simulink model "myrobot"  (R2019b)
settings: Solver=FixedStepAuto  StartTime=0.0  StopTime=2  FixedStep=0.001  MaxStep=0.005  RelTol=1e-3
undefined symbols (not defined in the file or in its folder): X, Y, Z
libraries: sm_lib x17, nesl_utility x13, robotmaniplib x4, simulink x2
(part 6 of 7)

== matlab function myrobot/TRAJECTORY GENERATION/MATLAB Function2 ==
  data: X output; Y output; Z output; T output; t input
function [X, Y, Z, T]  = trajectory_generator(t)

t = 0.1;
X = 0.3 + 0.2 * cos(5*pi*t);
Y = 0.45;
Z = 0.3 + 0.2 * sin(5*pi*t);

T = [1 0 0 X;
     0 1 0 Y;
     0 0 1 Z;
     0 0 0 1];

end

== matlab function myrobot/MATLAB Function ==
  data: q input; X output; Y output; Z output
function [X, Y, Z] = FK(q)

T_01 = [1 0 0 0;
        0 1 0 0;
        0 0 1 0.07;
        0 0 0 1]; 

T_1dot2 = [0 0 1 0.08;
           1 0 0 0;
           0 1 0 0.12;
           0 0 0 1];

T_2dot3 = [1 0 0 0;
           0 1 0 0.43;
           0 0 1 0;
           0 0 0 1];

T_3dot4 = [0 -1 0 0;
           0 0 1 0.335;
           -1 0 0 -0.08;
           0 0 0 1];

T_11dot = [cos(q(1)) -sin(q(1)) 0 0;
           sin(q(1)) cos(q(1)) 0 0;
           0 0 1 0
           0 0 0 1];

T_22dot = [cos(q(2)) -sin(q(2)) 0 0;
           sin(q(2)) cos(q(2)) 0 0;
           0 0 1 0
           0 0 0 1];

T_33dot = [cos(q(3)) -sin(q(3)) 0 0;
           sin(q(3)) cos(q(3)) 0 0;
           0 0 1 0
           0 0 0 1];

T_01dot = T_01 * T_11dot;
T_02dot = T_01dot * T_1dot2 * T_22dot;
T_03dot = T_02dot * T_2dot3 * T_33dot;
T_0EE = T_03dot * T_3dot4;


X = T_0EE(1,4);
Y = T_0EE(2,4);
Z = T_0EE(3,4);

end

== matlab function myrobot/MATLAB Function2 ==
  data: output output; q input; q_dot input; q_ddot input
function output = linear_parameterized(q, q_dot, q_ddot)

g = 9.81;

Y = [ q_dot(1)*q_dot(2)*sin(2*q(2)) - q_ddot(1)*(cos(2*q(2))/2 - 1/2), q_ddot(1)*sin(2*q(2)) + 2*q_dot(1)*q_dot(2)*cos(2*q(2)), q_dot(1)*((q_dot(2)*sin(2*q(2) + 2*q(3)))/2 + (q_dot(3)*sin(2*q(2) + 2*q(3)))/2) - q_ddot(1)*(cos(2*q(2) + 2*q(3))/2 - 1/2) + (q_dot(1)*q_dot(2)*sin(2*q(2) + 2*q(3)))/2 + (q_dot(1)*q_dot(3)*sin(2*q(2) + 2*q(3)))/2, q_ddot(1)*(cos(2*q(2))/2 + 1/2) - q_dot(1)*q_dot(2)*sin(2*q(2)), cos(q(2))*q_dot(2)^2 + q_ddot(2)*sin(q(2)), q_ddot(1)*sin(2*q(2) + 2*q(3)) + q_dot(1)*(q_dot(2)*cos(2*q(2) + 2*q(3)) + q_dot(3)*cos(2*q(2) + 2*q(3))) + q_dot(1)*q_dot(2)*cos(2*q(2) + 2*q(3)) + q_dot(1)*q_dot(3)*cos(2*q(2) + 2*q(3)), q_ddot(1), - sin(q(2))*q_dot(2)^2 + q_ddot(2)*cos(q(2)), q_ddot(1)*(cos(2*q(2) + 2*q(3))/2 + 1/2) - q_dot(1)*((q_dot(2)*sin(2*q(2) + 2*q(3)))/2 + (q_dot(3)*sin(2*q(2) + 2*q(3)))/2) - (q_dot(1)*q_dot(2)*sin(2*q(2) + 2*q(3)))/2 - (q_dot(1)*q_dot(3)*sin(2*q(2) + 2*q(3)))/2, q_dot(2)*(q_dot(2)*cos(q(2) + q(3)) + q_dot(3)*cos(q(2) + q(3))) + q_dot(3)*(q_dot(2)*cos(q(2) + q(3)) + q_dot(3)*cos(q(2) + q(3))) + q_ddot(2)*sin(q(2) + q(3)) + q_ddot(3)*sin(q(2) + q(3)),           0, q_ddot(2)*cos(q(2) + q(3)) - q_dot(3)*(q_dot(2)*sin(q(2) + q(3)) + q_dot(3)*sin(q(2) + q(3))) - q_dot(2)*(q_dot(2)*sin(q(2) + q(3)) + q_dot(3)*sin(q(2) + q(3))) + q_ddot(3)*cos(q(2) + q(3)),                         0,              0,              0,                       0, q_ddot(1), q_ddot(1), q_dot(1)*q_dot(2)*sin(2*q(2)) - q_ddot(1)*(cos(2*q(2))/2 - 1/2), q_ddot(1), q_dot(1)*q_dot(2)*sin(2*q(2)) - q_ddot(1)*(cos(2*q(2))/2 - 1/2), q_ddot(1), q_dot(1)*((q_dot(2)*sin(2*q(2) + 2*q(3)))/2 + (q_dot(3)*sin(2*q(2) + 2*q(3)))/2) - q_ddot(1)*(cos(2*q(2) + 2*q(3))/2 - 1/2) + (q_dot(1)*q_dot(2)*sin(2*q(2) + 2*q(3)))/2 + (q_dot(1)*q_dot(3)*sin(2*q(2) + 2*q(3)))/2, q_ddot(1), sin(q(2))*q_dot(2)^2 - q_ddot(2)*cos(q(2)), sin(q(2))*q_dot(2)^2 - q_ddot(2)*cos(q(2)), 2*q_ddot(1), q_dot(2)*(q_dot(2)*sin(q(2) + q(3)) + q_dot(3)*sin(q(2) + q(3))) + q_dot(3)*(q_dot(2)*sin(q(2) + q(3)) + q_dot(3)*sin(q(2) + q(3))) - q_ddot(2)*cos(q(2) + q(3)) - q_ddot(3)*cos(q(2) + q(3)), 2*q_ddot(1), q_dot(1)*(q_dot(2)*sin(2*q(2) + q(3)) + q_dot(3)*(sin(2*q(2) + q(3))/2 - sin(q(3))/2)) - q_ddot(1)*(cos(2*q(2) + q(3)) - cos(q(3))) - q_dot(3)*((q_dot(1)*sin(q(3)))/2 - (q_dot(1)*sin(2*q(2) + q(3)))/2) + q_dot(1)*q_dot(2)*sin(2*q(2) + q(3)), sin(q(2))*q_dot(2)^2 - q_ddot(2)*cos(q(2)), sin(q(2))*q_dot(2)^2 - q_ddot(2)*cos(q(2)), q_dot(2)*(q_dot(2)*sin(q(2) + q(3)) + q_dot(3)*sin(q(2) + q(3))) + q_dot(3)*(q_dot(2)*sin(q(2) + q(3)) + q_dot(3)*sin(q(2) + q(3))) - q_ddot(2)*cos(q(2) + q(3)) - q_ddot(3)*cos(q(2) + q(3));
                                           -(q_dot(1)^2*sin(2*q(2)))/2,                                       -q_dot(1)^2*cos(2*q(2)),                                                                                                                                                                                                                -(q_dot(1)^2*sin(2*q(2) + 2*q(3)))/2,                                            (q_dot(1)^2*sin(2*q(2)))/2,                            q_ddot(1)*sin(q(2)),                                                                                                                                                                                          -q_dot(1)^2*cos(2*q(2) + 2*q(3)),           0,                              q_ddot(1)*cos(q(2)),                                                                                                                                                                                                                 (q_dot(1)^2*sin(2*q(2) + 2*q(3)))/2,                                                                                                                                                                                                      q_ddot(1)*sin(q(2) + q(3)), q_ddot(2),                                                                                                                                                                                                      q_ddot(1)*cos(q(2) + q(3)), q_ddot(2) + q_ddot(3), -g*sin(q(2)), -g*sin(q(2)), -g*sin(q(2) + q(3)),           0,           0,                              q_ddot(2) - (q_dot(1)^2*sin(2*q(2)))/2,           0,                              q_ddot(2) - (q_dot(1)^2*sin(2*q(2)))/2,           0,                                                                                                                                                                                     q_ddot(2) + q_ddot(3) - (q_dot(1)^2*sin(2*q(2) + 2*q(3)))/2,           0,                           -q_ddot(1)*cos(q(2)),                           -q_ddot(1)*cos(q(2)),             0,                                                                                                                                                                                                     -q_ddot(1)*cos(q(2) + q(3)),             0,                                                                                                           - sin(2*q(2) + q(3))*q_dot(1)^2 + 2*q_ddot(2)*cos(q(3)) + q_ddot(3)*cos(q(3)) - q_dot(3)*sin(q(3))*(q_dot(2) + q_dot(3)) - q_dot(2)*q_dot(3)*sin(q(3)),                           -q_ddot(1)*cos(q(2)),                           -q_ddot(1)*cos(q(2)),                                                                                                                                                                                                     -q_ddot(1)*cos(q(2) + q(3));
                                                                         0,                                                                 0,                                                                                                                                                                                                                -(q_dot(1)^2*sin(2*q(2) + 2*q(3)))/2,                                                                         0,                                                  0,                                                                                                                                                                                          -q_dot(1)^2*cos(2*q(2) + 2*q(3)),           0,                                                    0,                                                                                                                                                                                                                 (q_dot(1)^2*sin(2*q(2) + 2*q(3)))/2,                                                                                                                                                                                                      q_ddot(1)*sin(q(2) + q(3)),           0,                                                                                                                                                                                                      q_ddot(1)*cos(q(2) + q(3)), q_ddot(2) + q_ddot(3),              0,              0, -g*sin(q(2) + q(3)),           0,           0,                                                                         0,           0,                                                                         0,           0,                                                                                                                                                                                     q_ddot(2) + q_ddot(3) - (q_dot(1)^2*sin(2*q(2) + 2*q(3)))/2,           0,                                                  0,                                                  0,             0,                                                                                                                                                                                                     -q_ddot(1)*cos(q(2) + q(3)),             0,                                                                                                                                                                                 (sin(q(3))/2 - sin(2*q(2) + q(3))/2)*q_dot(1)^2 + sin(q(3))*q_dot(2)^2 + q_ddot(2)*cos(q(3)),                                                  0,                                                  0,                                                                                                                                                                                                     -q_ddot(1)*cos(q(2) + q(3))];

THETA = [0.253740000000000,1.41285000000000e-07,0.0754340000000000,0.0212824000000000,-7.13886000000000e-08,2.67415000000000e-08,0.00604953000000000,0.00499483000000000,0.0104250000000000,2.13561000000000e-09,0.247523000000000,0.00274946000000000,0.0744749000000000,2.21400980000000,1.73854678600000,0.622883338500000,0.0521152000000000,0.0329527040000000,0.952024214000000,0.000192286280344500,0.371183215904572,0.0688146654633342,0.0753533118750375,0.0294165347194417,0.177120784000000,0.139083742880000,0.0598856414640000,0.0498306670800000,-0.0311344561750400,0.267839835555000,-0.167347701940840,0.159821302798087,-0.0470811354471933];

output = Y * THETA';

end

== matlab function myrobot/VERIFYING PASSIVITY PARAMETER LINEARIZATION/MATLAB Function1 ==
  data: q input; output output; q_dot input; a input; v input
function output = passivity_linear_parameterized(q, q_dot, a, v)

g = 9.81;

Y = [ (q_dot(1)*v(2)*sin(2*q(2)))/2 - a(1)*(cos(2*q(2))/2 - 1/2) + (q_dot(2)*v(1)*sin(2*q(2)))/2, a(1)*sin(2*q(2)) + q_dot(1)*v(2)*cos(2*q(2)) + q_dot(2)*v(1)*cos(2*q(2)), v(1)*((q_dot(2)*sin(2*q(2) + 2*q(3)))/2 + (q_dot(3)*sin(2*q(2) + 2*q(3)))/2) - a(1)*(cos(2*q(2) + 2*q(3))/2 - 1/2) + (q_dot(1)*v(2)*sin(2*q(2) + 2*q(3)))/2 + (q_dot(1)*v(3)*sin(2*q(2) + 2*q(3)))/2, a(1)*(cos(2*q(2))/2 + 1/2) - (q_dot(1)*v(2)*sin(2*q(2)))/2 - (q_dot(2)*v(1)*sin(2*q(2)))/2, a(2)*sin(q(2)) + q_dot(2)*v(2)*cos(q(2)), a(1)*sin(2*q(2) + 2*q(3)) + v(1)*(q_dot(2)*cos(2*q(2) + 2*q(3)) + q_dot(3)*cos(2*q(2) + 2*q(3))) + q_dot(1)*v(2)*cos(2*q(2) + 2*q(3)) + q_dot(1)*v(3)*cos(2*q(2) + 2*q(3)), a(1), a(2)*cos(q(2)) - q_dot(2)*v(2)*sin(q(2)), a(1)*(cos(2*q(2) + 2*q(3))/2 + 1/2) - v(1)*((q_dot(2)*sin(2*q(2) + 2*q(3)))/2 + (q_dot(3)*sin(2*q(2) + 2*q(3)))/2) - (q_dot(1)*v(2)*sin(2*q(2) + 2*q(3)))/2 - (q_dot(1)*v(3)*sin(2*q(2) + 2*q(3)))/2, v(2)*(q_dot(2)*cos(q(2) + q(3)) + q_dot(3)*cos(q(2) + q(3))) + v(3)*(q_dot(2)*cos(q(2) + q(3)) + q_dot(3)*cos(q(2) + q(3))) + a(2)*sin(q(2) + q(3)) + a(3)*sin(q(2) + q(3)),  0, a(2)*cos(q(2) + q(3)) - v(3)*(q_dot(2)*sin(q(2) + q(3)) + q_dot(3)*sin(q(2) + q(3))) - v(2)*(q_dot(2)*sin(q(2) + q(3)) + q_dot(3)*sin(q(2) + q(3))) + a(3)*cos(q(2) + q(3)),       0,              0,              0,                       0, a(1), a(1), (q_dot(1)*v(2)*sin(2*q(2)))/2 - a(1)*(cos(2*q(2))/2 - 1/2) + (q_dot(2)*v(1)*sin(2*q(2)))/2, a(1), (q_dot(1)*v(2)*sin(2*q(2)))/2 - a(1)*(cos(2*q(2))/2 - 1/2) + (q_dot(2)*v(1)*sin(2*q(2)))/2, a(1), v(1)*((q_dot(2)*sin(2*q(2) + 2*q(3)))/2 + (q_dot(3)*sin(2*q(2) + 2*q(3)))/2) - a(1)*(cos(2*q(2) + 2*q(3))/2 - 1/2) + (q_dot(1)*v(2)*sin(2*q(2) + 2*q(3)))/2 + (q_dot(1)*v(3)*sin(2*q(2) + 2*q(3)))/2, a(1), q_dot(2)*v(2)*sin(q(2)) - a(2)*cos(q(2)), q_dot(2)*v(2)*sin(q(2)) - a(2)*cos(q(2)), 2*a(1), v(2)*(q_dot(2)*sin(q(2) + q(3)) + q_dot(3)*sin(q(2) + q(3))) + v(3)*(q_dot(2)*sin(q(2) + q(3)) + q_dot(3)*sin(q(2) + q(3))) - a(2)*cos(q(2) + q(3)) - a(3)*cos(q(2) + q(3)), 2*a(1), v(1)*(q_dot(2)*sin(2*q(2) + q(3)) + q_dot(3)*(sin(2*q(2) + q(3))/2 - sin(q(3))/2)) - a(1)*(cos(2*q(2) + q(3)) - cos(q(3))) - v(3)*((q_dot(1)*sin(q(3)))/2 - (q_dot(1)*sin(2*q(2) + q(3)))/2) + q_dot(1)*v(2)*sin(2*q(2) + q(3)), q_dot(2)*v(2)*sin(q(2)) - a(2)*cos(q(2)), q_dot(2)*v(2)*sin(q(2)) - a(2)*cos(q(2)), v(2)*(q_dot(2)*sin(q(2) + q(3)) + q_dot(3)*sin(q(2) + q(3))) + v(3)*(q_dot(2)*sin(q(2) + q(3)) + q_dot(3)*sin(q(2) + q(3))) - a(2)*cos(q(2) + q(3)) - a(3)*cos(q(2) + q(3));
                                                               -(q_dot(1)*v(1)*sin(2*q(2)))/2,                                                 -q_dot(1)*v(1)*cos(2*q(2)),                                                                                                                                                                              -(q_dot(1)*v(1)*sin(2*q(2) + 2*q(3)))/2,                                                                (q_dot(1)*v(1)*sin(2*q(2)))/2,                             a(1)*sin(q(2)),                                                                                                                                                        -q_dot(1)*v(1)*cos(2*q(2) + 2*q(3)),  0,                             a(1)*cos(q(2)),                                                                                                                                                                               (q_dot(1)*v(1)*sin(2*q(2) + 2*q(3)))/2,                                                                                                                                                                             a(1)*sin(q(2) + q(3)), a(2),                                                                                                                                                                             a(1)*cos(q(2) + q(3)), a(2) + a(3), -g*sin(q(2)), -g*sin(q(2)), -g*sin(q(2) + q(3)),  0,  0,                                                           a(2) - (q_dot(1)*v(1)*sin(2*q(2)))/2,  0,                                                           a(2) - (q_dot(1)*v(1)*sin(2*q(2)))/2,  0,                                                                                                                                                                     a(2) + a(3) - (q_dot(1)*v(1)*sin(2*q(2) + 2*q(3)))/2,  0,                            -a(1)*cos(q(2)),                            -a(1)*cos(q(2)),    0,                                                                                                                                                                            -a(1)*cos(q(2) + q(3)),    0,                                                                                                             2*a(2)*cos(q(3)) + a(3)*cos(q(3)) - v(3)*sin(q(3))*(q_dot(2) + q_dot(3)) - q_dot(3)*v(2)*sin(q(3)) - q_dot(1)*v(1)*sin(2*q(2) + q(3)),                            -a(1)*cos(q(2)),                            -a(1)*cos(q(2)),                                                                                                                                                                            -a(1)*cos(q(2) + q(3));
                                                                                              0,                                                                            0,                                                                                                                                                                              -(q_dot(1)*v(1)*sin(2*q(2) + 2*q(3)))/2,                                                                                              0,                                          0,                                                                                                                                                        -q_dot(1)*v(1)*cos(2*q(2) + 2*q(3)),  0,                                          0,                                                                                                                                                                               (q_dot(1)*v(1)*sin(2*q(2) + 2*q(3)))/2,                                                                                                                                                                             a(1)*sin(q(2) + q(3)),  0,                                                                                                                                                                             a(1)*cos(q(2) + q(3)), a(2) + a(3),              0,              0, -g*sin(q(2) + q(3)),  0,  0,                                                                                              0,  0,                                                                                              0,  0,                                                                                                                                                                     a(2) + a(3) - (q_dot(1)*v(1)*sin(2*q(2) + 2*q(3)))/2,  0,                                          0,                                          0,    0,                                                                                                                                                                            -a(1)*cos(q(2) + q(3)),    0,                                                                                                                                                       a(2)*cos(q(3)) + q_dot(2)*v(2)*sin(q(3)) - q_dot(1)*v(1)*(sin(2*q(2) + q(3))/2 - sin(q(3))/2),                                          0,                                          0,                                                                                                                                                                            -a(1)*cos(q(2) + q(3))];
 
THETA = [0.253740000000000,1.41285000000000e-07,0.0754340000000000,0.0212824000000000,-7.13886000000000e-08,2.67415000000000e-08,0.00604953000000000,0.00499483000000000,0.0104250000000000,2.13561000000000e-09,0.247523000000000,0.00274946000000000,0.0744749000000000,2.21400980000000,1.73854678600000,0.622883338500000,0.0521152000000000,0.0329527040000000,0.952024214000000,0.000192286280344500,0.371183215904572,0.0688146654633342,0.0753533118750375,0.0294165347194417,0.177120784000000,0.139083742880000,0.0598856414640000,0.0498306670800000,-0.0311344561750400,0.267839835555000,-0.167347701940840,0.159821302798087,-0.0470811354471933];

output = Y * THETA';

end

== matlab function myrobot/JOINT SPACE PASSIVITY BASED ROBUST CONTROLLER/MATLAB Function3 ==
  data: q input; output output; q_dot input; a input; v input; delta_theta input
function output = robust_passivity_linear_parameterized(q, q_dot, a, v, delta_theta)

g = 9.81;

Y = [ (q_dot(1)*v(2)*sin(2*q(2)))/2 - a(1)*(cos(2*q(2))/2 - 1/2) + (q_dot(2)*v(1)*sin(2*q(2)))/2, a(1)*sin(2*q(2)) + q_dot(1)*v(2)*cos(2*q(2)) + q_dot(2)*v(1)*cos(2*q(2)), v(1)*((q_dot(2)*sin(2*q(2) + 2*q(3)))/2 + (q_dot(3)*sin(2*q(2) + 2*q(3)))/2) - a(1)*(cos(2*q(2) + 2*q(3))/2 - 1/2) + (q_dot(1)*v(2)*sin(2*q(2) + 2*q(3)))/2 + (q_dot(1)*v(3)*sin(2*q(2) + 2*q(3)))/2, a(1)*(cos(2*q(2))/2 + 1/2) - (q_dot(1)*v(2)*sin(2*q(2)))/2 - (q_dot(2)*v(1)*sin(2*q(2)))/2, a(2)*sin(q(2)) + q_dot(2)*v(2)*cos(q(2)), a(1)*sin(2*q(2) + 2*q(3)) + v(1)*(q_dot(2)*cos(2*q(2) + 2*q(3)) + q_dot(3)*cos(2*q(2) + 2*q(3))) + q_dot(1)*v(2)*cos(2*q(2) + 2*q(3)) + q_dot(1)*v(3)*cos(2*q(2) + 2*q(3)), a(1), a(2)*cos(q(2)) - q_dot(2)*v(2)*sin(q(2)), a(1)*(cos(2*q(2) + 2*q(3))/2 + 1/2) - v(1)*((q_dot(2)*sin(2*q(2) + 2*q(3)))/2 + (q_dot(3)*sin(2*q(2) + 2*q(3)))/2) - (q_dot(1)*v(2)*sin(2*q(2) + 2*q(3)))/2 - (q_dot(1)*v(3)*sin(2*q(2) + 2*q(3)))/2, v(2)*(q_dot(2)*cos(q(2) + q(3)) + q_dot(3)*cos(q(2) + q(3))) + v(3)*(q_dot(2)*cos(q(2) + q(3)) + q_dot(3)*cos(q(2) + q(3))) + a(2)*sin(q(2) + q(3)) + a(3)*sin(q(2) + q(3)),  0, a(2)*cos(q(2) + q(3)) - v(3)*(q_dot(2)*sin(q(2) + q(3)) + q_dot(3)*sin(q(2) + q(3))) - v(2)*(q_dot(2)*sin(q(2) + q(3)) + q_dot(3)*sin(q(2) + q(3))) + a(3)*cos(q(2) + q(3)),       0,              0,              0,                       0, a(1), a(1), (q_dot(1)*v(2)*sin(2*q(2)))/2 - a(1)*(cos(2*q(2))/2 - 1/2) + (q_dot(2)*v(1)*sin(2*q(2)))/2, a(1), (q_dot(1)*v(2)*sin(2*q(2)))/2 - a(1)*(cos(2*q(2))/2 - 1/2) + (q_dot(2)*v(1)*sin(2*q(2)))/2, a(1), v(1)*((q_dot(2)*sin(2*q(2) + 2*q(3)))/2 + (q_dot(3)*sin(2*q(2) + 2*q(3)))/2) - a(1)*(cos(2*q(2) + 2*q(3))/2 - 1/2) + (q_dot(1)*v(2)*sin(2*q(2) + 2*q(3)))/2 + (q_dot(1)*v(3)*sin(2*q(2) + 2*q(3)))/2, a(1), q_dot(2)*v(2)*sin(q(2)) - a(2)*cos(q(2)), q_dot(2)*v(2)*sin(q(2)) - a(2)*cos(q(2)), 2*a(1), v(2)*(q_dot(2)*sin(q(2) + q(3)) + q_dot(3)*sin(q(2) + q(3))) + v(3)*(q_dot(2)*sin(q(2) + q(3)) + q_dot(3)*sin(q(2) + q(3))) - a(2)*cos(q(2) + q(3)) - a(3)*cos(q(2) + q(3)), 2*a(1), v(1)*(q_dot(2)*sin(2*q(2) + q(3)) + q_dot(3)*(sin(2*q(2) + q(3))/2 - sin(q(3))/2)) - a(1)*(cos(2*q(2) + q(3)) - cos(q(3))) - v(3)*((q_dot(1)*sin(q(3)))/2 - (q_dot(1)*sin(2*q(2) + q(3)))/2) + q_dot(1)*v(2)*sin(2*q(2) + q(3)), q_dot(2)*v(2)*sin(q(2)) - a(2)*cos(q(2)), q_dot(2)*v(2)*sin(q(2)) - a(2)*cos(q(2)), v(2)*(q_dot(2)*sin(q(2) + q(3)) + q_dot(3)*sin(q(2) + q(3))) + v(3)*(q_dot(2)*sin(q(2) + q(3)) + q_dot(3)*sin(q(2) + q(3))) - a(2)*cos(q(2) + q(3)) - a(3)*cos(q(2) + q(3));
                                                               -(q_dot(1)*v(1)*sin(2*q(2)))/2,                                                 -q_dot(1)*v(1)*cos(2*q(2)),                                                                                                                                                                              -(q_dot(1)*v(1)*sin(2*q(2) + 2*q(3)))/2,                                                                (q_dot(1)*v(1)*sin(2*q(2)))/2,                             a(1)*sin(q(2)),                                                                                                                                                        -q_dot(1)*v(1)*cos(2*q(2) + 2*q(3)),  0,                             a(1)*cos(q(2)),                                                                                                                                                                               (q_dot(1)*v(1)*sin(2*q(2) + 2*q(3)))/2,                                                                                                                                                                             a(1)*sin(q(2) + q(3)), a(2),                                                                                                                                                                             a(1)*cos(q(2) + q(3)), a(2) + a(3), -g*sin(q(2)), -g*sin(q(2)), -g*sin(q(2) + q(3)),  0,  0,                                                           a(2) - (q_dot(1)*v(1)*sin(2*q(2)))/2,  0,                                                           a(2) - (q_dot(1)*v(1)*sin(2*q(2)))/2,  0,                                                                                                                                                                     a(2) + a(3) - (q_dot(1)*v(1)*sin(2*q(2) + 2*q(3)))/2,  0,                            -a(1)*cos(q(2)),                            -a(1)*cos(q(2)),    0,                                                                                                                                                                            -a(1)*cos(q(2) + q(3)),    0,                                                                                                             2*a(2)*cos(q(3)) + a(3)*cos(q(3)) - v(3)*sin(q(3))*(q_dot(2) + q_dot(3)) - q_dot(3)*v(2)*sin(q(3)) - q_dot(1)*v(1)*sin(2*q(2) + q(3)),                            -a(1)*cos(q(2)),                            -a(1)*cos(q(2)),                                                                                                                                                                            -a(1)*cos(q(2) + q(3));
                                                                                              0,                                                                            0,                                                                                                                                                                              -(q_dot(1)*v(1)*sin(2*q(2) + 2*q(3)))/2,                                                                                              0,                                          0,                                                                                                                                                        -q_dot(1)*v(1)*cos(2*q(2) + 2*q(3)),  0,                                          0,                                                                                                                                                                               (q_dot(1)*v(1)*sin(2*q(2) + 2*q(3)))/2,                                                                                                                                                                             a(1)*sin(q(2) + q(3)),  0,                                                                                                                                                                             a(1)*cos(q(2) + q(3)), a(2) + a(3),              0,              0, -g*sin(q(2) + q(3)),  0,  0,                                                                                              0,  0,                                                                                              0,  0,                                                                                                                                                                     a(2) + a(3) - (q_dot(1)*v(1)*sin(2*q(2) + 2*q(3)))/2,  0,                                          0,                                          0,    0,                                                                                                                                                                            -a(1)*cos(q(2) + q(3)),    0,                                                                                                                                                       a(2)*cos(q(3)) + q_dot(2)*v(2)*sin(q(3)) - q_dot(1)*v(1)*(sin(2*q(2) + q(3))/2 - sin(q(3))/2),                                          0,                                          0,                                                                                                                                                                            -a(1)*cos(q(2) + q(3))];
 
THETA = [0.253740000000000,1.41285000000000e-07,0.0754340000000000,0.0212824000000000,-7.13886000000000e-08,2.67415000000000e-08,0.00604953000000000,0.00499483000000000,0.0104250000000000,2.13561000000000e-09,0.247523000000000,0.00274946000000000,0.0744749000000000,2.21400980000000,1.73854678600000,0.622883338500000,0.0521152000000000,0.0329527040000000,0.952024214000000,0.000192286280344500,0.371183215904572,0.0688146654633342,0.0753533118750375,0.0294165347194417,0.177120784000000,0.139083742880000,0.0598856414640000,0.0498306670800000,-0.0311344561750400,0.267839835555000,-0.167347701940840,0.159821302798087,-0.0470811354471933];

output = Y * (THETA' + delta_theta);

end

== matlab function myrobot/JOINT SPACE PASSIVITY BASED ROBUST CONTROLLER/MATLAB Function1 ==
  data: q input; q_dot input; a input; v input; r input; delta_theta output
function delta_theta = calc_delta_theta(q, q_dot, a, v, r)
    g = 9.81;
    
    %----- PARAMETER TO TUNE -----%
    epsilon = 0.1;
    rho = 1;
    %-----------------------------%
    Y = [ (q_dot(1)*v(2)*sin(2*q(2)))/2 - a(1)*(cos(2*q(2))/2 - 1/2) + (q_dot(2)*v(1)*sin(2*q(2)))/2, a(1)*sin(2*q(2)) + q_dot(1)*v(2)*cos(2*q(2)) + q_dot(2)*v(1)*cos(2*q(2)), v(1)*((q_dot(2)*sin(2*q(2) + 2*q(3)))/2 + (q_dot(3)*sin(2*q(2) + 2*q(3)))/2) - a(1)*(cos(2*q(2) + 2*q(3))/2 - 1/2) + (q_dot(1)*v(2)*sin(2*q(2) + 2*q(3)))/2 + (q_dot(1)*v(3)*sin(2*q(2) + 2*q(3)))/2, a(1)*(cos(2*q(2))/2 + 1/2) - (q_dot(1)*v(2)*sin(2*q(2)))/2 - (q_dot(2)*v(1)*sin(2*q(2)))/2, a(2)*sin(q(2)) + q_dot(2)*v(2)*cos(q(2)), a(1)*sin(2*q(2) + 2*q(3)) + v(1)*(q_dot(2)*cos(2*q(2) + 2*q(3)) + q_dot(3)*cos(2*q(2) + 2*q(3))) + q_dot(1)*v(2)*cos(2*q(2) + 2*q(3)) + q_dot(1)*v(3)*cos(2*q(2) + 2*q(3)), a(1), a(2)*cos(q(2)) - q_dot(2)*v(2)*sin(q(2)), a(1)*(cos(2*q(2) + 2*q(3))/2 + 1/2) - v(1)*((q_dot(2)*sin(2*q(2) + 2*q(3)))/2 + (q_dot(3)*sin(2*q(2) + 2*q(3)))/2) - (q_dot(1)*v(2)*sin(2*q(2) + 2*q(3)))/2 - (q_dot(1)*v(3)*sin(2*q(2) + 2*q(3)))/2, v(2)*(q_dot(2)*cos(q(2) + q(3)) + q_dot(3)*cos(q(2) + q(3))) + v(3)*(q_dot(2)*cos(q(2) + q(3)) + q_dot(3)*cos(q(2) + q(3))) + a(2)*sin(q(2) + q(3)) + a(3)*sin(q(2) + q(3)),  0, a(2)*cos(q(2) + q(3)) - v(3)*(q_dot(2)*sin(q(2) + q(3)) + q_dot(3)*sin(q(2) + q(3))) - v(2)*(q_dot(2)*sin(q(2) + q(3)) + q_dot(3)*sin(q(2) + q(3))) + a(3)*cos(q(2) + q(3)),       0,              0,              0,                       0, a(1), a(1), (q_dot(1)*v(2)*sin(2*q(2)))/2 - a(1)*(cos(2*q(2))/2 - 1/2) + (q_dot(2)*v(1)*sin(2*q(2)))/2, a(1), (q_dot(1)*v(2)*sin(2*q(2)))/2 - a(1)*(cos(2*q(2))/2 - 1/2) + (q_dot(2)*v(1)*sin(2*q(2)))/2, a(1), v(1)*((q_dot(2)*sin(2*q(2) + 2*q(3)))/2 + (q_dot(3)*sin(2*q(2) + 2*q(3)))/2) - a(1)*(cos(2*q(2) + 2*q(3))/2 - 1/2) + (q_dot(1)*v(2)*sin(2*q(2) + 2*q(3)))/2 + (q_dot(1)*v(3)*sin(2*q(2) + 2*q(3)))/2, a(1), q_dot(2)*v(2)*sin(q(2)) - a(2)*cos(q(2)), q_dot(2)*v(2)*sin(q(2)) - a(2)*cos(q(2)), 2*a(1), v(2)*(q_dot(2)*sin(q(2) + q(3)) + q_dot(3)*sin(q(2) + q(3))) + v(3)*(q_dot(2)*sin(q(2) + q(3)) + q_dot(3)*sin(q(2) + q(3))) - a(2)*cos(q(2) + q(3)) - a(3)*cos(q(2) + q(3)), 2*a(1), v(1)*(q_dot(2)*sin(2*q(2) + q(3)) + q_dot(3)*(sin(2*q(2) + q(3))/2 - sin(q(3))/2)) - a(1)*(cos(2*q(2) + q(3)) - cos(q(3))) - v(3)*((q_dot(1)*sin(q(3)))/2 - (q_dot(1)*sin(2*q(2) + q(3)))/2) + q_dot(1)*v(2)*sin(2*q(2) + q(3)), q_dot(2)*v(2)*sin(q(2)) - a(2)*cos(q(2)), q_dot(2)*v(2)*sin(q(2)) - a(2)*cos(q(2)), v(2)*(q_dot(2)*sin(q(2) + q(3)) + q_dot(3)*sin(q(2) + q(3))) + v(3)*(q_dot(2)*sin(q(2) + q(3)) + q_dot(3)*sin(q(2) + q(3))) - a(2)*cos(q(2) + q(3)) - a(3)*cos(q(2) + q(3));
                                                               -(q_dot(1)*v(1)*sin(2*q(2)))/2,                                                 -q_dot(1)*v(1)*cos(2*q(2)),                                                                                                                                                                              -(q_dot(1)*v(1)*sin(2*q(2) + 2*q(3)))/2,                                                                (q_dot(1)*v(1)*sin(2*q(2)))/2,                             a(1)*sin(q(2)),                                                                                                                                                        -q_dot(1)*v(1)*cos(2*q(2) + 2*q(3)),  0,                             a(1)*cos(q(2)),                                                                                                                                                                               (q_dot(1)*v(1)*sin(2*q(2) + 2*q(3)))/2,                                                                                                                                                                             a(1)*sin(q(2) + q(3)), a(2),                                                                                                                                                                             a(1)*cos(q(2) + q(3)), a(2) + a(3), -g*sin(q(2)), -g*sin(q(2)), -g*sin(q(2) + q(3)),  0,  0,                                                           a(2) - (q_dot(1)*v(1)*sin(2*q(2)))/2,  0,                                                           a(2) - (q_dot(1)*v(1)*sin(2*q(2)))/2,  0,                                                                                                                                                                     a(2) + a(3) - (q_dot(1)*v(1)*sin(2*q(2) + 2*q(3)))/2,  0,                            -a(1)*cos(q(2)),                            -a(1)*cos(q(2)),    0,                                                                                                                                                                            -a(1)*cos(q(2) + q(3)),    0,                                                                                                             2*a(2)*cos(q(3)) + a(3)*cos(q(3)) - v(3)*sin(q(3))*(q_dot(2) + q_dot(3)) - q_dot(3)*v(2)*sin(q(3)) - q_dot(1)*v(1)*sin(2*q(2) + q(3)),                            -a(1)*cos(q(2)),                            -a(1)*cos(q(2)),                                                                                                                                                                            -a(1)*cos(q(2) + q(3));
                                                                                              0,                                                                            0,                                                                                                                                                                              -(q_dot(1)*v(1)*sin(2*q(2) + 2*q(3)))/2,                                                                                              0,                                          0,                                                                                                                                                        -q_dot(1)*v(1)*cos(2*q(2) + 2*q(3)),  0,                                          0,                                                                                                                                                                               (q_dot(1)*v(1)*sin(2*q(2) + 2*q(3)))/2,                                                                                                                                                                             a(1)*sin(q(2) + q(3)),  0,                                                                                                                                                                             a(1)*cos(q(2) + q(3)), a(2) + a(3),              0,              0, -g*sin(q(2) + q(3)),  0,  0,                                                                                              0,  0,                                                                                              0,  0,                                                                                                                                                                     a(2) + a(3) - (q_dot(1)*v(1)*sin(2*q(2) + 2*q(3)))/2,  0,                                          0,                                          0,    0,                                                                                                                                                                            -a(1)*cos(q(2) + q(3)),    0,                                                                                                                                                       a(2)*cos(q(3)) + q_dot(2)*v(2)*sin(q(3)) - q_dot(1)*v(1)*(sin(2*q(2) + q(3))/2 - sin(q(3))/2),                                          0,                                          0,                                                                                                                                                                            -a(1)*cos(q(2) + q(3))];
    value = Y'*r;
    if (norm(value) > epsilon)
        delta_theta = -rho * (value / norm(value));
    else
        delta_theta = -rho / epsilon * value;
    end
end

== matlab function myrobot/JOINT SPACE PASSIVITY BASED ADAPTIVE CONTROLLER/MATLAB Function4 ==
  data: updated_theta output; q input; output output; q_dot input; a input; v input; estimated_theta_dot input; updated_theta input
function [updated_theta,output] = adaptive_passivity_linear_parameterized(q, q_dot, a, v, estimated_theta_dot, updated_theta)

g = 9.81;

Y = [ (q_dot(1)*v(2)*sin(2*q(2)))/2 - a(1)*(cos(2*q(2))/2 - 1/2) + (q_dot(2)*v(1)*sin(2*q(2)))/2, a(1)*sin(2*q(2)) + q_dot(1)*v(2)*cos(2*q(2)) + q_dot(2)*v(1)*cos(2*q(2)), v(1)*((q_dot(2)*sin(2*q(2) + 2*q(3)))/2 + (q_dot(3)*sin(2*q(2) + 2*q(3)))/2) - a(1)*(cos(2*q(2) + 2*q(3))/2 - 1/2) + (q_dot(1)*v(2)*sin(2*q(2) + 2*q(3)))/2 + (q_dot(1)*v(3)*sin(2*q(2) + 2*q(3)))/2, a(1)*(cos(2*q(2))/2 + 1/2) - (q_dot(1)*v(2)*sin(2*q(2)))/2 - (q_dot(2)*v(1)*sin(2*q(2)))/2, a(2)*sin(q(2)) + q_dot(2)*v(2)*cos(q(2)), a(1)*sin(2*q(2) + 2*q(3)) + v(1)*(q_dot(2)*cos(2*q(2) + 2*q(3)) + q_dot(3)*cos(2*q(2) + 2*q(3))) + q_dot(1)*v(2)*cos(2*q(2) + 2*q(3)) + q_dot(1)*v(3)*cos(2*q(2) + 2*q(3)), a(1), a(2)*cos(q(2)) - q_dot(2)*v(2)*sin(q(2)), a(1)*(cos(2*q(2) + 2*q(3))/2 + 1/2) - v(1)*((q_dot(2)*sin(2*q(2) + 2*q(3)))/2 + (q_dot(3)*sin(2*q(2) + 2*q(3)))/2) - (q_dot(1)*v(2)*sin(2*q(2) + 2*q(3)))/2 - (q_dot(1)*v(3)*sin(2*q(2) + 2*q(3)))/2, v(2)*(q_dot(2)*cos(q(2) + q(3)) + q_dot(3)*cos(q(2) + q(3))) + v(3)*(q_dot(2)*cos(q(2) + q(3)) + q_dot(3)*cos(q(2) + q(3))) + a(2)*sin(q(2) + q(3)) + a(3)*sin(q(2) + q(3)),  0, a(2)*cos(q(2) + q(3)) - v(3)*(q_dot(2)*sin(q(2) + q(3)) + q_dot(3)*sin(q(2) + q(3))) - v(2)*(q_dot(2)*sin(q(2) + q(3)) + q_dot(3)*sin(q(2) + q(3))) + a(3)*cos(q(2) + q(3)),       0,              0,              0,                       0, a(1), a(1), (q_dot(1)*v(2)*sin(2*q(2)))/2 - a(1)*(cos(2*q(2))/2 - 1/2) + (q_dot(2)*v(1)*sin(2*q(2)))/2, a(1), (q_dot(1)*v(2)*sin(2*q(2)))/2 - a(1)*(cos(2*q(2))/2 - 1/2) + (q_dot(2)*v(1)*sin(2*q(2)))/2, a(1), v(1)*((q_dot(2)*sin(2*q(2) + 2*q(3)))/2 + (q_dot(3)*sin(2*q(2) + 2*q(3)))/2) - a(1)*(cos(2*q(2) + 2*q(3))/2 - 1/2) + (q_dot(1)*v(2)*sin(2*q(2) + 2*q(3)))/2 + (q_dot(1)*v(3)*sin(2*q(2) + 2*q(3)))/2, a(1), q_dot(2)*v(2)*sin(q(2)) - a(2)*cos(q(2)), q_dot(2)*v(2)*sin(q(2)) - a(2)*cos(q(2)), 2*a(1), v(2)*(q_dot(2)*sin(q(2) + q(3)) + q_dot(3)*sin(q(2) + q(3))) + v(3)*(q_dot(2)*sin(q(2) + q(3)) + q_dot(3)*sin(q(2) + q(3))) - a(2)*cos(q(2) + q(3)) - a(3)*cos(q(2) + q(3)), 2*a(1), v(1)*(q_dot(2)*sin(2*q(2) + q(3)) + q_dot(3)*(sin(2*q(2) + q(3))/2 - sin(q(3))/2)) - a(1)*(cos(2*q(2) + q(3)) - cos(q(3))) - v(3)*((q_dot(1)*sin(q(3)))/2 - (q_dot(1)*sin(2*q(2) + q(3)))/2) + q_dot(1)*v(2)*sin(2*q(2) + q(3)), q_dot(2)*v(2)*sin(q(2)) - a(2)*cos(q(2)), q_dot(2)*v(2)*sin(q(2)) - a(2)*cos(q(2)), v(2)*(q_dot(2)*sin(q(2) + q(3)) + q_dot(3)*sin(q(2) + q(3))) + v(3)*(q_dot(2)*sin(q(2) + q(3)) + q_dot(3)*sin(q(2) + q(3))) - a(2)*cos(q(2) + q(3)) - a(3)*cos(q(2) + q(3));
                                                               -(q_dot(1)*v(1)*sin(2*q(2)))/2,                                                 -q_dot(1)*v(1)*cos(2*q(2)),                                                                                                                                                                              -(q_dot(1)*v(1)*sin(2*q(2) + 2*q(3)))/2,                                                                (q_dot(1)*v(1)*sin(2*q(2)))/2,                             a(1)*sin(q(2)),                                                                                                                                                        -q_dot(1)*v(1)*cos(2*q(2) + 2*q(3)),  0,                             a(1)*cos(q(2)),                                                                                                                                                                               (q_dot(1)*v(1)*sin(2*q(2) + 2*q(3)))/2,                                                                                                                                                                             a(1)*sin(q(2) + q(3)), a(2),                                                                                                                                                                             a(1)*cos(q(2) + q(3)), a(2) + a(3), -g*sin(q(2)), -g*sin(q(2)), -g*sin(q(2) + q(3)),  0,  0,                                                           a(2) - (q_dot(1)*v(1)*sin(2*q(2)))/2,  0,                                                           a(2) - (q_dot(1)*v(1)*sin(2*q(2)))/2,  0,                                                                                                                                                                     a(2) + a(3) - (q_dot(1)*v(1)*sin(2*q(2) + 2*q(3)))/2,  0,                            -a(1)*cos(q(2)),                            -a(1)*cos(q(2)),    0,                                                                                                                                                                            -a(1)*cos(q(2) + q(3)),    0,                                                                                                             2*a(2)*cos(q(3)) + a(3)*cos(q(3)) - v(3)*sin(q(3))*(q_dot(2) + q_dot(3)) - q_dot(3)*v(2)*sin(q(3)) - q_dot(1)*v(1)*sin(2*q(2) + q(3)),                            -a(1)*cos(q(2)),                            -a(1)*cos(q(2)),                                                                                                                                                                            -a(1)*cos(q(2) + q(3));
                                                                                              0,                                                                            0,                                                                                                                                                                              -(q_dot(1)*v(1)*sin(2*q(2) + 2*q(3)))/2,                                                                                              0,                                          0,                                                                                                                                                        -q_dot(1)*v(1)*cos(2*q(2) + 2*q(3)),  0,                                          0,                                                                                                                                                                               (q_dot(1)*v(1)*sin(2*q(2) + 2*q(3)))/2,                                                                                                                                                                             a(1)*sin(q(2) + q(3)),  0,                                                                                                                                                                             a(1)*cos(q(2) + q(3)), a(2) + a(3),              0,              0, -g*sin(q(2) + q(3)),  0,  0,                                                                                              0,  0,                                                                                              0,  0,                                                                                                                                                                     a(2) + a(3) - (q_dot(1)*v(1)*sin(2*q(2) + 2*q(3)))/2,  0,                                          0,                                          0,    0,                                                                                                                                                                            -a(1)*cos(q(2) + q(3)),    0,                                                                                                                                                       a(2)*cos(q(3)) + q_dot(2)*v(2)*sin(q(3)) - q_dot(1)*v(1)*(sin(2*q(2) + q(3))/2 - sin(q(3))/2),                                          0,                                          0,                                                                                                                                                                            -a(1)*cos(q(2) + q(3))];
 
updated_theta = updated_theta + estimated_theta_dot * 0.001;
output = Y * updated_theta;
end
